simulink model "bouncing_int"  (R2021a)
settings: Solver=VariableStepAuto  StartTime=0.0  StopTime=time_sim*2  RelTol=1e-5
values from neighbouring files (symbols this model uses):
  e_coeff = 0.3    [run.m]
  f = 0.04    [run.m]
  I = eye(3).*(0.4*m*r_bouncer^2)    [run.m]
  m = 1    [run.m]
  r_bouncer = 0.1    [run.m]
  w = 50*2*pi/(24*3600)    (= 0.00363610260832)    [run.m]
libraries: vrlib x4, simulink x2, aerolibutil x1
settings Model: Creator=danie  LastModifiedBy=danie
settings SolverCC: ZeroCrossAlgorithm=Adaptive
settings DebuggingCC: IgnoredZcDiagnostic=none

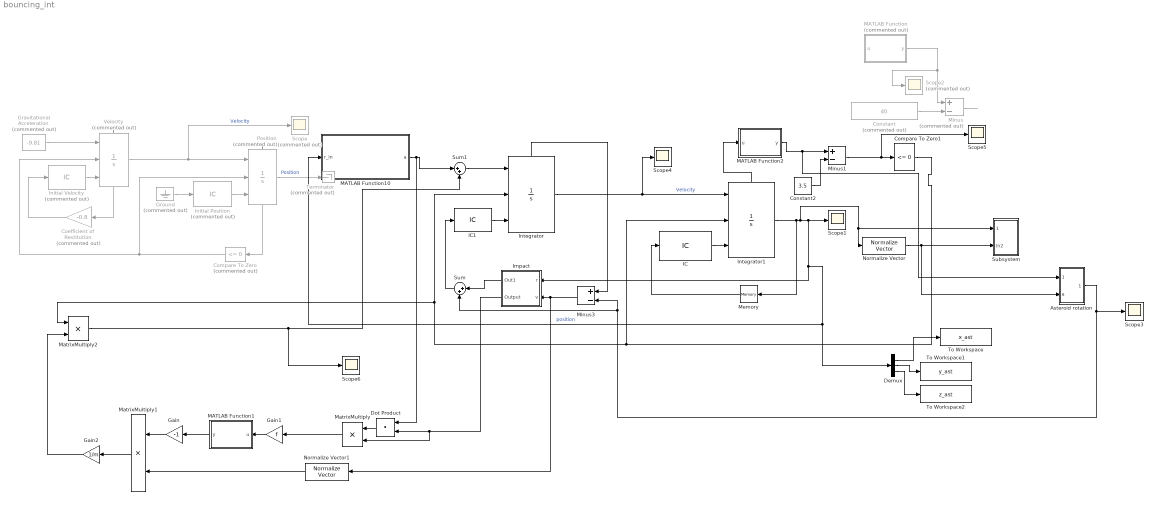
== system bouncing_int ==
  Asteroid rotation : Subsystem
  Coefficient of Restitution : Gain  Commented=on  Gain=-0.8  SaturateOnIntegerOverflow=on  OutDataTypeStr=Inherit: Same as input  ParamDataTypeStr=Inherit: Same as input
  Compare To Zero1 : simulink/Logic and Bit Operations/Compare To Zero  relop=<=  OutDataTypeStr=boolean
  Compare To Zero : simulink/Logic and Bit Operations/Compare To Zero  Commented=on  relop=<=  OutDataTypeStr=boolean
  Constant : Constant  Commented=on  Value=40
  Constant2 : Constant  Value=3.5
  Demux : Demux  Outputs=3
  Dot Product : DotProduct  InputSameDT=on  OutDataTypeStr=Inherit: Inherit via internal rule
  Gain : Gain  Gain=-1
  Gain1 : Gain  Gain=f
  Gain2 : Gain  Gain=1/m
  Gravitational Acceleration : Constant  Commented=on  Value=-9.81
  Ground : Ground  Commented=on
  IC : InitialCondition  Value=[-13.5;0;0]
  IC1 : InitialCondition  Value=[0;0;0]
  Impact : Subsystem
  Initial Position : InitialCondition  Commented=on  Value=10
  Initial Velocity : InitialCondition  Commented=on  Value=15
  Integrator : Integrator  ExternalReset=rising  InitialConditionSource=external  ShowStatePort=on
  Integrator1 : Integrator  ExternalReset=rising  InitialConditionSource=external  ShowStatePort=on
  MATLAB Function : MATLAB Function  Commented=on  TreatAsAtomicUnit=on
  MATLAB Function1 : MATLAB Function  TreatAsAtomicUnit=on
  MATLAB Function10 : MATLAB Function  TreatAsAtomicUnit=on
  MATLAB Function2 : MATLAB Function  TreatAsAtomicUnit=on
  MatrixMultiply : Product
  MatrixMultiply1 : Product
  MatrixMultiply2 : Product
  Memory : Memory
  Minus : Sum  Commented=on  Inputs=+-
  Minus1 : Sum  Inputs=+-
  Minus3 : Sum  Inputs=+-
  Normalize Vector : vrlib/Utilities/Normalize Vector  maxzero=0
  Normalize Vector1 : vrlib/Utilities/Normalize Vector  maxzero=0
  Position : Integrator  Commented=on  ExternalReset=rising  InitialConditionSource=external  LimitOutput=on  LowerSaturationLimit=0  ShowStatePort=on
  Scope : Scope  Commented=on
  Scope{1,3..6} (5 alike) : Scope
  Scope2 : Scope  Commented=on
  Subsystem : Subsystem
  Sum : Sum  Inputs=|++
  Sum1 : Sum  Inputs=|++
  Terminator : Terminator  Commented=on
  To Workspace : ToWorkspace  VariableName=x_ast  SaveFormat=Timeseries  SampleTime=-1
  To Workspace1 : ToWorkspace  VariableName=y_ast  SaveFormat=Timeseries  SampleTime=-1
  To Workspace2 : ToWorkspace  VariableName=z_ast  SaveFormat=Timeseries  SampleTime=-1
  Velocity : Integrator  Commented=on  ExternalReset=rising  InitialConditionSource=external  ShowStatePort=on
  wires:
  Velocity/State -> Coefficient of Restitution/1
  Initial Velocity/1 -> Velocity/3
  Gravitational Acceleration/1 -> Velocity/1
  Compare To Zero/1 -> Velocity/2, Position/2
  Ground/1 -> Initial Position/1
  Position/1 -> Terminator/1  "Position"
  Velocity/1 -> Scope/1, Position/1  "Velocity"
  Position/State -> Compare To Zero/1
  Coefficient of Restitution/1 -> Initial Velocity/1
  Initial Position/1 -> Position/3
  Integrator/1 -> Scope4/1, Integrator1/1  "Velocity"
  IC/1 -> Integrator1/3
  IC1/1 -> Integrator/3
  Integrator1/1 -> Memory/1, Normalize Vector/1, Subsystem/1(position), Demux/1, MATLAB Function10/1(r_in), Impact/1(r), Scope1/1  "position"
  Constant/1 -> Minus/2
  Minus/1 -> ?
  MATLAB Function/1(y) -> Scope2/1, Minus/1
  Minus1/1 -> Scope5/1, Compare To Zero1/1
  Constant2/1 -> Minus1/2
  Memory/1 -> IC/1
  Compare To Zero1/1 -> Integrator/2, MatrixMultiply2/1, Integrator1/2
  Integrator1/State -> MATLAB Function2/1(u)
  MATLAB Function2/1(y) -> Asteroid rotation/1(In1), Minus1/1
  Normalize Vector/1 -> Subsystem/2(In2), Asteroid rotation/2(a)
  Integrator/State -> Minus3/1
  Asteroid rotation/1(Out1) -> Scope3/1, Minus3/2, Sum/2
  Minus3/1 -> Normalize Vector1/1, Impact/2(v)
  Demux/1 -> To Workspace/1
  Demux/2 -> To Workspace1/1
  Demux/3 -> To Workspace2/1
  Impact/1(Out1) -> Sum/1
  Sum/1 -> IC1/1
  Impact/2(Output) -> MatrixMultiply/2, Dot Product/2
  MATLAB Function10/1(a) -> Sum1/1, Dot Product/1
  Dot Product/1 -> MatrixMultiply/1
  MatrixMultiply/1 -> Gain1/1
  Gain1/1 -> MATLAB Function1/1(u)
  Normalize Vector1/1 -> MatrixMultiply1/2
  MATLAB Function1/1(y) -> Gain/1
  Gain/1 -> MatrixMultiply1/1
  MatrixMultiply1/1 -> Gain2/1
  Gain2/1 -> MatrixMultiply2/2
  Sum1/1 -> Integrator/1
  MatrixMultiply2/1 -> Scope6/1, Sum1/2

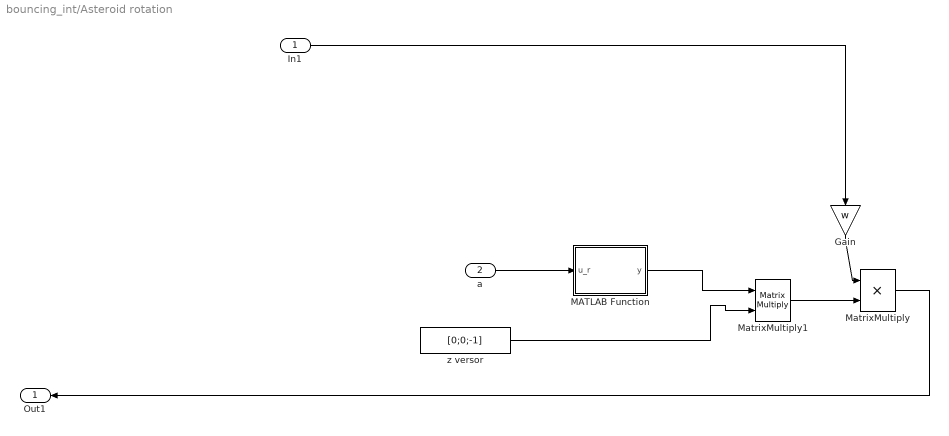
== system bouncing_int/Asteroid rotation ==
  In1 : Inport
  a : Inport  Port=2
  Gain : Gain  Gain=w
  MATLAB Function : MATLAB Function  TreatAsAtomicUnit=on
  MatrixMultiply : Product
  MatrixMultiply1 : Product  Multiplication=Matrix(*)
  z versor : Constant  Value=[0;0;-1]
  Out1 : Outport
  wires:
  In1/1 -> Gain/1
  Gain/1 -> MatrixMultiply/1
  MatrixMultiply1/1 -> MatrixMultiply/2
  MatrixMultiply/1 -> Out1/1
  z versor/1 -> MatrixMultiply1/2
  a/1 -> MATLAB Function/1(u_r)
  MATLAB Function/1(y) -> MatrixMultiply1/1

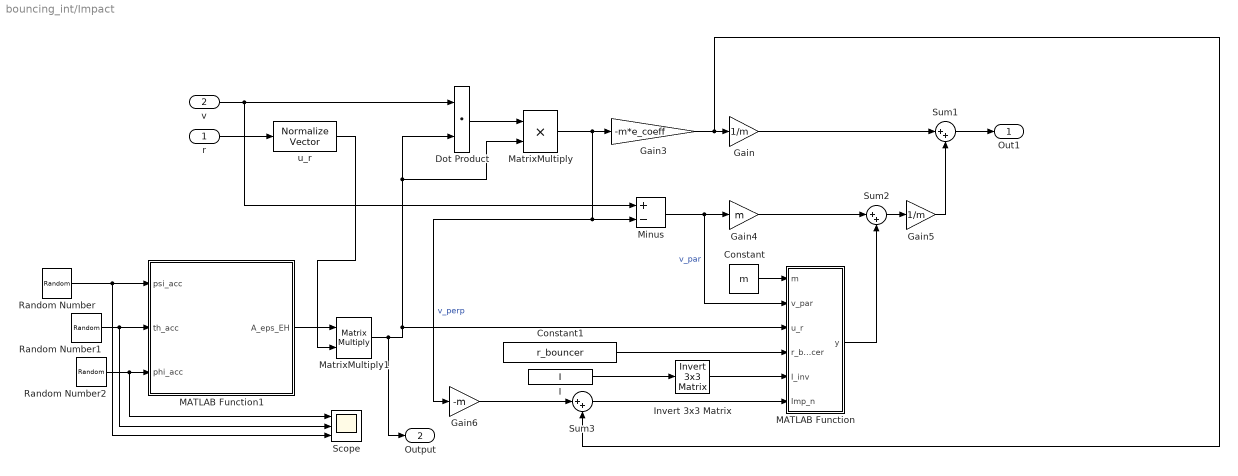
== system bouncing_int/Impact ==
  r : Inport
  v : Inport  Port=2
  Constant : Constant  Value=m
  Constant1 : Constant  Value=r_bouncer
  Dot Product : DotProduct  InputSameDT=on  OutDataTypeStr=Inherit: Inherit via internal rule
  Gain : Gain  Gain=1/m
  Gain3 : Gain  Gain=-m*e_coeff
  Gain4 : Gain  Gain=m
  Gain5 : Gain  Gain=1/m
  Gain6 : Gain  Gain=-m
  I : Constant  Value=I
  Invert 3x3 Matrix : aerolibutil/Invert  3x3 Matrix
  MATLAB Function : MATLAB Function  TreatAsAtomicUnit=on
  MATLAB Function1 : MATLAB Function  TreatAsAtomicUnit=on
  MatrixMultiply : Product
  MatrixMultiply1 : Product  Multiplication=Matrix(*)
  Minus : Sum  Inputs=+-
  Random Number : RandomNumber  Variance=0.0034  SampleTime=0.1
  Random Number1 : RandomNumber  Variance=0.0034  Seed=1  SampleTime=0.1
  Random Number2 : RandomNumber  Variance=0.0034  Seed=2  SampleTime=0.1
  Scope : Scope  NumInputPorts=3
  Sum1 : Sum  Inputs=|++
  Sum2 : Sum  Inputs=|++
  Sum3 : Sum  Inputs=|++
  u_r : vrlib/Utilities/Normalize Vector  maxzero=0
  Out1 : Outport
  Output : Outport  Port=2
  wires:
  Gain3/1 -> Gain/1, Sum3/2
  Dot Product/1 -> MatrixMultiply/1
  Invert 3x3 Matrix/1 -> MATLAB Function/5(I_inv)
  MatrixMultiply/1 -> Gain6/1, Minus/2, Gain3/1  "v_perp"
  Minus/1 -> MATLAB Function/2(v_par), Gain4/1  "v_par"
  MATLAB Function/1(y) -> Sum2/2
  Sum2/1 -> Gain5/1
  Constant/1 -> MATLAB Function/1(m)
  r/1 -> u_r/1
  Gain5/1 -> Sum1/2
  Constant1/1 -> MATLAB Function/4(r_bouncer)
  Gain6/1 -> Sum3/1
  Sum3/1 -> MATLAB Function/6(Imp_n)
  Sum1/1 -> Out1/1
  I/1 -> Invert 3x3 Matrix/1
  Gain/1 -> Sum1/1
  v/1 -> Dot Product/1, Minus/1
  u_r/1 -> MatrixMultiply1/2
  Gain4/1 -> Sum2/1
  MATLAB Function1/1(A_eps_EH) -> MatrixMultiply1/1
  MatrixMultiply1/1 -> Output/1, MatrixMultiply/2, Dot Product/2, MATLAB Function/3(u_r)
  Random Number/1 -> Scope/3, MATLAB Function1/1(psi_acc)
  Random Number2/1 -> Scope/1, MATLAB Function1/3(phi_acc)
  Random Number1/1 -> Scope/2, MATLAB Function1/2(th_acc)

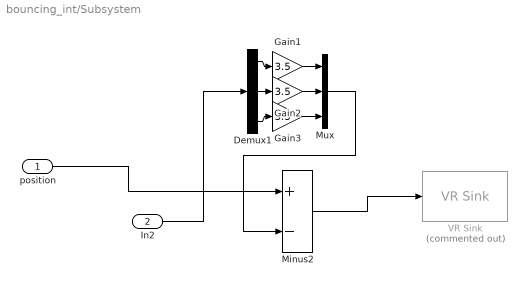
== system bouncing_int/Subsystem ==
  position : Inport
  In2 : Inport  Port=2
  Demux1 : Demux  Outputs=3
  Gain1 : Gain  Gain=3.5
  Gain2 : Gain  Gain=3.5
  Gain3 : Gain  Gain=3.5
  Minus2 : Sum  Inputs=+-
  Mux : Mux  Inputs=3
  VR Sink : vrlib/VR Sink  Commented=on  InstantiateOnLoad=on  SampleTime=0.1  ViewEnable=on  RemoteChange=off  RemoteView=off  FieldsWritten=STLEXP_Transform.translation.3.1.1.double  WorldFileName=ito_bounce.x3d  AutoView=off  VideoDimensions=[]  AllowVariableSize=off
  wires:
  Minus2/1 -> VR Sink/1
  Demux1/2 -> Gain2/1
  Gain2/1 -> Mux/2
  Demux1/1 -> Gain1/1
  Demux1/3 -> Gain3/1
  Mux/1 -> Minus2/2
  Gain1/1 -> Mux/1
  Gain3/1 -> Mux/3
  position/1 -> Minus2/1
  In2/1 -> Demux1/1

== matlab function bouncing_int/Impact/MATLAB Function ==
  data: m input; y output; v_par input; u_r input; r_bouncer input; I_inv input; Imp_n input
function y = fcn(m,v_par,u_r,r_bouncer,I_inv,Imp_n)
if norm(v_par)==0
    y=[0;0;0];
else
% y=-min([norm(m*v_par)/norm(cross(u_r,eye(3)+m*r_bouncer^2*I_inv)*(cross(u_r,v_par/norm(v_par)))),Imp_n])*v_par/norm(v_par);
y=-min([norm(m*v_par)/norm([0 -u_r(3) u_r(2); u_r(3) 0 -u_r(1); -u_r(2) u_r(1) 0]*(eye(3)+m*r_bouncer^2*I_inv)*(cross(u_r,v_par/norm(v_par)))),norm(Imp_n)])*v_par/norm(v_par);

end

== matlab function bouncing_int/MATLAB Function ==
  data: u input; y output
function y = fcn(u)

y = norm(u(:));

== matlab function bouncing_int/MATLAB Function2 ==
  data: u input; y output
function y = fcn(u)

y = norm(u(:));

== matlab function bouncing_int/Asteroid rotation/MATLAB Function ==
  data: u_r input; y output
function y = fcn(u_r)
y=[0 -u_r(3) u_r(2); u_r(3) 0 -u_r(1); -u_r(2) u_r(1) 0];

== matlab function bouncing_int/Impact/MATLAB Function1 ==
  data: psi_acc input; A_eps_EH output; th_acc input; phi_acc input
function A_eps_EH = fcn(psi_acc,th_acc,phi_acc)
A_eps_EH = [cos(psi_acc)*cos(th_acc)  (cos(psi_acc)*sin(th_acc)*sin(phi_acc)+sin(psi_acc)*cos(phi_acc)) (-cos(psi_acc)*sin(th_acc)*cos(phi_acc)+sin(psi_acc)*sin(phi_acc));
                -sin(psi_acc)*cos(th_acc) (-sin(psi_acc)*sin(th_acc)*sin(phi_acc)+cos(psi_acc)*cos(phi_acc))  (sin(psi_acc)*sin(th_acc)*cos(phi_acc)+cos(psi_acc)*sin(phi_acc));
                 sin(th_acc)               -cos(th_acc)*sin(phi_acc)                                           cos(th_acc)*cos(phi_acc)];

== matlab function bouncing_int/MATLAB Function1 ==
  data: u input; y output
function y = fcn(u)

y = norm(u(:));

== matlab function bouncing_int/MATLAB Function10 ==
  data: r_in input; a output
function a  = asteroid_gravity_point_model(r_in)
G=6.674e-11; %m3/(kg*s2)
mass= 1.7952e+05; %LOW 2009TD17 %2.090805433926013e+08;%kg%Bennu
mu=mass*G;
r_=[r_in(1),r_in(2),r_in(3)];
r=norm(r_);
a=((-mu*r_/(r^3)))'; %m/s^2
